simulink model "HJI_sliding_mode"  (R2019b)
settings: Solver=VariableStepAuto  StartTime=0.0  StopTime=10  RelTol=1e-3
settings Model: Creator=Alien  LastModifiedBy=Alien

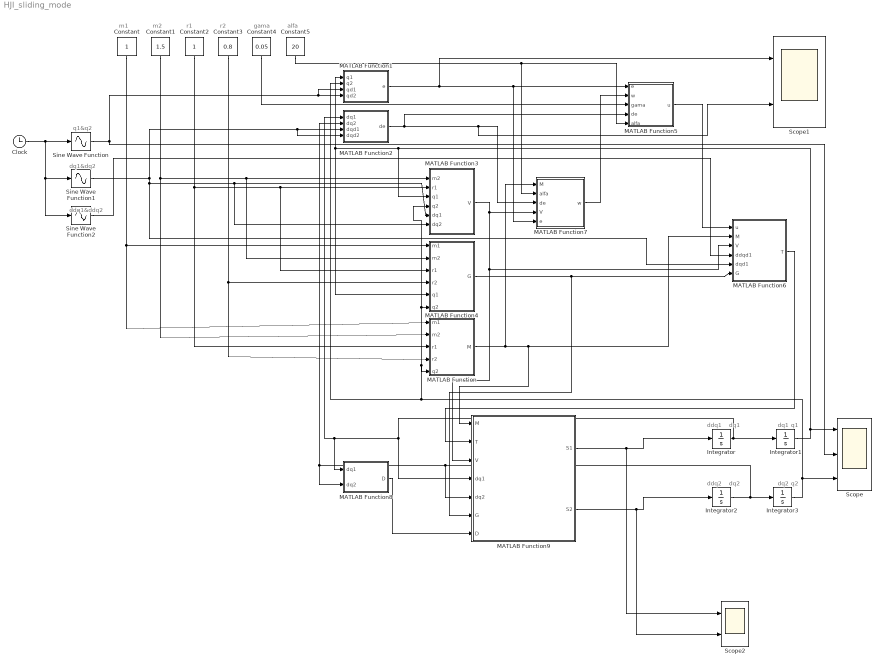
== system HJI_sliding_mode ==
  note: ddq1
  note: dq1
  note: dq1
  note: q1
  note: dq1&dq2
  note: q1&q2
  note: m1
  note: m2
  note: r1
  note: r2
  note: alfa
  note: gama
  note: ddq1&ddq2
  note: ddq2
  note: dq2
  note: q2
  note: dq2
  Clock : Clock
  Constant : Constant
  Constant1 : Constant  Value=1.5
  Constant2 : Constant
  Constant3 : Constant  Value=0.8
  Constant4 : Constant  Value=0.05
  Constant5 : Constant  Value=20
  Integrator : Integrator  InitialCondition=2
  Integrator1 : Integrator  InitialCondition=1
  Integrator2 : Integrator  InitialCondition=3
  Integrator3 : Integrator  InitialCondition=2
  MATLAB Function : MATLAB Function  TreatAsAtomicUnit=on
  MATLAB Function1 : MATLAB Function  TreatAsAtomicUnit=on
  MATLAB Function2 : MATLAB Function  TreatAsAtomicUnit=on
  MATLAB Function3 : MATLAB Function  TreatAsAtomicUnit=on
  MATLAB Function4 : MATLAB Function  TreatAsAtomicUnit=on
  MATLAB Function5 : MATLAB Function  TreatAsAtomicUnit=on
  MATLAB Function6 : MATLAB Function  TreatAsAtomicUnit=on
  MATLAB Function7 : MATLAB Function  TreatAsAtomicUnit=on
  MATLAB Function8 : MATLAB Function  TreatAsAtomicUnit=on
  MATLAB Function9 : MATLAB Function  TreatAsAtomicUnit=on
  Scope : Scope  NumInputPorts=3
  Scope1 : Scope  NumInputPorts=2
  Scope2 : Scope  NumInputPorts=2
  Sine Wave Function : Sin  TimeSource=Use external signal  SampleTime=0
  Sine Wave Function1 : Sin  TimeSource=Use external signal  Phase=pi/2  SampleTime=0
  Sine Wave Function2 : Sin  TimeSource=Use external signal  Amplitude=-1  SampleTime=0
  wires:
  Clock/1 -> Sine Wave Function2/1, Sine Wave Function1/1, Sine Wave Function/1
  Sine Wave Function1/1 -> MATLAB Function2/4(dqd2), MATLAB Function2/3(dqd1), MATLAB Function6/5(dqd1), MATLAB Function3/6(dq2), MATLAB Function3/5(dq1)
  Sine Wave Function2/1 -> MATLAB Function6/4(ddqd1)
  Constant1/1 -> MATLAB Function/2(m2), MATLAB Function4/2(m2), MATLAB Function3/1(m2)
  Constant2/1 -> MATLAB Function/3(r1), MATLAB Function4/3(r1), MATLAB Function3/2(r1)
  Constant/1 -> MATLAB Function4/1(m1), MATLAB Function/1(m1)
  Constant3/1 -> MATLAB Function/4(r2), MATLAB Function4/4(r2)
  MATLAB Function/1(M) -> MATLAB Function9/1(M), MATLAB Function6/2(M), MATLAB Function7/1(M)
  Constant5/1 -> MATLAB Function5/5(alfa), MATLAB Function7/2(alfa)
  MATLAB Function2/1(de) -> MATLAB Function5/4(de), Scope1/2, MATLAB Function7/3(de)
  MATLAB Function1/1(e) -> Scope1/1, MATLAB Function5/1(e), MATLAB Function7/5(e)
  MATLAB Function3/1(V) -> MATLAB Function9/3(V), MATLAB Function6/3(V), MATLAB Function7/4(V)
  MATLAB Function7/1(w) -> MATLAB Function5/2(w)
  Constant4/1 -> MATLAB Function5/3(gama)
  MATLAB Function5/1(u) -> MATLAB Function6/1(u)
  MATLAB Function4/1(G) -> MATLAB Function9/6(G), MATLAB Function6/6(G)
  Integrator/1 -> Integrator1/1, MATLAB Function9/4(dq1), MATLAB Function8/1(dq1), MATLAB Function2/1(dq1)
  Integrator2/1 -> MATLAB Function8/2(dq2), MATLAB Function2/2(dq2), MATLAB Function9/5(dq2), Integrator3/1
  Integrator1/1 -> Scope/1, MATLAB Function3/3(q1), MATLAB Function4/5(q1), MATLAB Function1/1(q1)
  Integrator3/1 -> Scope/3, MATLAB Function3/4(q2), MATLAB Function4/6(q2), MATLAB Function/5(q2), MATLAB Function1/2(q2)
  MATLAB Function8/1(D) -> MATLAB Function9/7(D)
  MATLAB Function6/1(T) -> MATLAB Function9/2(T)
  MATLAB Function9/1(S1) -> Scope2/1, Integrator/1
  MATLAB Function9/2(S2) -> Scope2/2, Integrator2/1
  Sine Wave Function/1 -> Scope/2, MATLAB Function1/3(qd1), MATLAB Function1/4(qd2)

== matlab function HJI_sliding_mode/MATLAB Function1 ==
  data: q1 input; e output size=[2 1]; q2 input; qd1 input; qd2 input
function e = fcn(q1, q2, qd1, qd2)
e1 = q1 - qd1;
e2 = q2 - qd2;

e = [e1 e2]';

== matlab function HJI_sliding_mode/MATLAB Function ==
  data: m1 input; M output size=[2 2]; m2 input; r1 input; r2 input; q2 input
function M = fcn(m1, m2, r1, r2, q2)
M11 = (m1 + m2) * r1^2 + m2 * r2^2 + 2 * m2 * r1 * r2 *cos(q2);
M22 = m2 * r2^2;
M21 = m2 * r2^2 + m2 * r1 * r2 * cos(q2);
M12 = M21;
M = [M11 M12;M21 M22];

== matlab function HJI_sliding_mode/MATLAB Function2 ==
  data: dq1 input; de output size=[2 1]; dq2 input; dqd1 input; dqd2 input
function de = fcn(dq1, dq2, dqd1, dqd2)
de1 = dq1 - dqd1;
de2 = dq2 - dqd2;

de = [de1 de2]';

== matlab function HJI_sliding_mode/MATLAB Function3 ==
  data: m2 input; V output size=[2 2]; r1 input; q1 input; q2 input; dq1 input; dq2 input
function V = fcn(m2, r1, q1, q2, dq1, dq2)
vt = m2 * r1 * q2;
v11 = -dq2 * vt;
v12 = -vt * (dq1 + dq2);
v21 = q1 * vt;
v22 = 0;

V = [v11 v12;v21 v22];

== matlab function HJI_sliding_mode/MATLAB Function4 ==
  data: m1 input; G output; m2 input; r1 input; r2 input; q1 input; q2 input
function G = fcn(m1, m2, r1, r2, q1, q2)
g1 = (m1 + m2) * r1 * cos(q2) + m2 * r2 * cos(q1 + q2);
g2 = m2 * r2 * cos(q1 + q2);

G = [g1;g2];

== matlab function HJI_sliding_mode/MATLAB Function5 ==
  data: e input; u output size=[2 1]; w input; gama input; de input; alfa input
function u = fcn(e, w, gama, de, alfa)
u = -e - w - 0.5 * 1/gama^2 * (de + alfa *e);

== matlab function HJI_sliding_mode/MATLAB Function6 ==
  data: u input; T output size=[2 1]; M input; V input; ddqd1 input; dqd1 input; G input
function T = fcn(u, M, V, ddqd1, dqd1, G)
ddqd = [ddqd1 ddqd1]';
dqd = [dqd1 dqd1]';

T = u + M * ddqd + V * dqd + G;

== matlab function HJI_sliding_mode/MATLAB Function7 ==
  data: M input; w output size=[2 1]; alfa input; de input; V input; e input
function w = fcn(M, alfa, de, V, e)
w = M * alfa * de + V * alfa * e;

== matlab function HJI_sliding_mode/MATLAB Function8 ==
  data: dq1 input; D output size=[2 1]; dq2 input
function D = fcn(dq1, dq2)
d1 = 10 * dq1 + 30 * sign(dq1);
d2 = 10 * dq2 + 30 * sign(dq2);

D = [d1;d2];

== matlab function HJI_sliding_mode/MATLAB Function9 ==
  data: M input; S1 output; T input; V input; dq1 input; dq2 input; G input; D input; S2 output
function [S1, S2] = fcn(M, T, V, dq1, dq2, G, D)
S = inv(M) * (T - V * [dq1;dq2] - G - D);
S1 = S(1);
S2 = S(2);
